simulink model "Experiment2JessDelPath_cs"  (Simulink 9.0)
settings: Solver=ode5  StartTime=0.0  StopTime=inf  FixedStep=1/300  RelTol=1e-3
PreLoadFcn:
  | mbxruntime.callbacks.PreLoadFcn(bdroot);
PostLoadFcn:
  | mbxruntime.callbacks.PostLoadFcn(bdroot);
InitFcn:
  | mbxruntime.callbacks.InitFcn(bdroot);
StartFcn:
  | mbxruntime.callbacks.StartFcn(bdroot);
StopFcn:
  | mbxruntime.callbacks.StopFcn(bdroot);
undefined symbols (not defined in the file or in its folder): DiscIntNeverNeededParam, InitImageOutputDir
libraries: PreScanSimulinkLibrary x84, simulink x43, simulink_extras x20, dspnetwork x2, vrlib x1
(part 14 of 14)

== system Experiment2JessDelPath_cs/Audi_A8_Sedan_1/Dynamics_Simple_3D/Chassis/Bicycle_model_[XYZ]/RoadContact/RoadGeometry/zRR_lowerpenetrationdetph ==
  penetrationdepth : Inport
  position_z : Inport  Port=2
  normal_z : Inport  Port=3
  Add : Sum  Inputs=-+
  Configurable Subsystem : Subsystem  BlockChoice=Discrete Transfer Fcn  mask{ComputationMode=ComputationMode}
      mask prompts: ComputationMode "Compuation mode:"
      mask init:
      | SetComputationMode(gcb,ComputationMode);
      settings: AttributesFormatString=%<BlockChoice>  OpenFcn=BringToFront(gcb);  MemberBlocks=Discrete Transfer Fcn,Transfer Fcn
      settings: TemplateBlock=|
      | PreScanSimulinkLibrary/Configurable Subsystems/TransferFunction
      | lowerpenetrationdetph/Configurable
      | Subsystem
  Constant : Constant  Value=Inf
  Constant1 : Constant  Value=-6
  Constant2 : Constant  Value=-Inf
  Data Type Conversion : DataTypeConversion  OutDataTypeStr=double
  MinMax : MinMax
  Product : Product  RndMeth=Zero
  Product1 : Product  Inputs=/*  RndMeth=Zero
  Product2 : Product  RndMeth=Zero
  Rate Limiter Dynamic : simulink/Discontinuities/Rate Limiter Dynamic
      settings: SourceProductName=Simulink
  Relational Operator : RelationalOperator  Operator===  OutDataTypeStr=boolean  RndMeth=Nearest
  Sum of Elements : Sum  Inputs=+
  Sum of Elements1 : Sum  Inputs=+
  Sum of Elements2 : Sum  Inputs=+
  Switch : Switch
  z : Outport
  wires:
  Configurable Subsystem/1(Out1) -> z/1
  Rate Limiter Dynamic/1 -> Configurable Subsystem/1(In1)
  Switch/1 -> Rate Limiter Dynamic/3
  Constant2/1 -> Switch/3
  Constant1/1 -> Switch/1
  Sum of Elements2/1 -> Switch/2
  Constant/1 -> Rate Limiter Dynamic/1
  Product1/1 -> Rate Limiter Dynamic/2
  position_z/1 -> Add/2
  Product2/1 -> Add/1
  Sum of Elements/1 -> Product1/2
  Sum of Elements1/1 -> Product1/1
  Relational Operator/1 -> Data Type Conversion/1
  Product/1 -> Sum of Elements/1
  MinMax/1 -> Relational Operator/2
  penetrationdepth/1 -> Sum of Elements2/1, Relational Operator/1, MinMax/1, Product2/1
  Add/1 -> Product/2
  normal_z/1 -> Product2/2
  Data Type Conversion/1 -> Sum of Elements1/1, Product/1

== system Experiment2JessDelPath_cs/Audi_A8_Sedan_1/Dynamics_Simple_3D/Chassis/Bicycle_model_[XYZ]/RoadContact/RoadGeometry/zRR_tyreinfo ==
  In1 : Inport
  Bus Selector2 : BusSelector  OutputSignals=TireRR.cp0.penetrationdepth,TireRR.cp1.penetrationdepth,TireRR.cp2.penetrationdepth,TireRR.cp3.penetrationdepth,TireRR.cp0.position.z,TireRR.cp1.position.z,TireRR.cp2.position.z,TireRR.cp3.position.z,TireRR.cp0.normal.z,TireRR.cp1.normal.z,TireRR.cp2.normal.z,TireRR.cp3.normal.z
  Mux11 : Mux
  Mux12 : Mux
  Mux13 : Mux
  penetrationdepth : Outport
  position_z : Outport  Port=2
  normal_z : Outport  Port=3
  wires:
  Mux13/1 -> normal_z/1
  Mux12/1 -> position_z/1
  Mux11/1 -> penetrationdepth/1
  In1/1 -> Bus Selector2/1
  Bus Selector2/12 -> Mux13/4  "<z>"
  Bus Selector2/11 -> Mux13/3  "<z>"
  Bus Selector2/10 -> Mux13/2  "<z>"
  Bus Selector2/9 -> Mux13/1  "<z>"
  Bus Selector2/8 -> Mux12/4  "<z>"
  Bus Selector2/7 -> Mux12/3  "<z>"
  Bus Selector2/6 -> Mux12/2  "<z>"
  Bus Selector2/5 -> Mux12/1  "<z>"
  Bus Selector2/4 -> Mux11/4  "<penetrationdepth>"
  Bus Selector2/3 -> Mux11/3  "<penetrationdepth>"
  Bus Selector2/2 -> Mux11/2  "<penetrationdepth>"
  Bus Selector2/1 -> Mux11/1  "<penetrationdepth>"

== system Experiment2JessDelPath_cs/Audi_A8_Sedan_1/Dynamics_Simple_3D/Chassis/Bicycle_model_[XYZ]/X_Motion/Max RPM and zero- velocity detection/Configurable Subsystem ==
  Discrete Step : Step  Time=0.0001  Before=1  After=0  SampleTime=TimeStep
  Out1 : Outport
  wires:
  Discrete Step/1 -> Out1/1

== system Experiment2JessDelPath_cs/Audi_A8_Sedan_1/Dynamics_Simple_3D/Chassis/Bicycle_model_[XYZ]/X_Motion/Max RPM and zero- velocity detection/SR-Memory ==
  Signal : Inport
  Set : Inport  Port=2
  Reset : Inport  Port=3
  Constant : Constant  Value=0
  Detect Rise Positive : simulink/Logic and Bit Operations/Detect Rise Positive  vinit=0  InputProcessing=Inherited  OutDataTypeStr=uint8
  Detect Rise Positive1 : simulink/Logic and Bit Operations/Detect Rise Positive  vinit=0  InputProcessing=Inherited  OutDataTypeStr=uint8
  Manual Switch : ManualSwitch
  Manual Switch1 : ManualSwitch
  Switch : Switch  Criteria=u2 ~= 0
  Switch1 : Switch  Criteria=u2 ~= 0
  Unit Delay : UnitDelay  SampleTime=-1
  Out : Outport
  wires:
  Manual Switch/1 -> Switch/2
  Detect Rise Positive/1 -> Manual Switch/1
  Set/1 -> Manual Switch/2, Detect Rise Positive/1
  Unit Delay/1 -> Switch/3
  Signal/1 -> Switch/1
  Detect Rise Positive1/1 -> Manual Switch1/1
  Reset/1 -> Detect Rise Positive1/1, Manual Switch1/2
  Manual Switch1/1 -> Switch1/2
  Switch1/1 -> Out/1, Unit Delay/1
  Switch/1 -> Switch1/3
  Constant/1 -> Switch1/1

== system Experiment2JessDelPath_cs/Audi_A8_Sedan_1/PreScan_Contact_Sensor/Vehicle Local to World/state2FullState/limit roll/Substitute 90 & 270 deg (and its plurals)/Angle 0-360 deg limiter ==
  Angle [deg] : Inport
  Gain : Gain  Gain=1/360
  Gain1 : Gain  Gain=360
  Rounding Function : Rounding
  Sum : Sum  Inputs=|-+
  LimAngle [deg] : Outport
  wires:
  Gain/1 -> Rounding Function/1
  Rounding Function/1 -> Gain1/1
  Gain1/1 -> Sum/1
  Angle [deg]/1 -> Gain/1, Sum/2
  Sum/1 -> LimAngle [deg]/1

== system Experiment2JessDelPath_cs/Audi_A8_Sedan_1/Dynamics_Simple_3D/Chassis/Bicycle_model_[XYZ]/RoadContact/RoadGeometry/Calc_z/zC ==
  Array : Inport
  Compare To Constant : simulink/Logic and Bit Operations/Compare To Constant  relop=>  const=0  OutDataTypeStr=uint8  ZeroCross=off
  Constant : Constant  Value=NaN
  Product : Product  Inputs=*/  RndMeth=Zero
  Sum of Elements : Sum  Inputs=+
  Switch : Switch
  Width : Width
  Mean : Outport
  wires:
  Array/1 -> Sum of Elements/1, Width/1
  Sum of Elements/1 -> Product/1
  Width/1 -> Product/2, Compare To Constant/1
  Compare To Constant/1 -> Switch/2
  Product/1 -> Switch/1
  Constant/1 -> Switch/3
  Switch/1 -> Mean/1

== system Experiment2JessDelPath_cs/Audi_A8_Sedan_1/Dynamics_Simple_3D/Chassis/Bicycle_model_[XYZ]/RoadContact/RoadGeometry/zFL_lowerpenetrationdetph/Configurable Subsystem ==
  In1 : Inport
  Discrete Transfer Fcn : DiscreteTransferFcn  Numerator="[  1-exp(-( ( TimeStep ) / (1/(2*pi)) ) )  ]"  Denominator="[  1   -exp(-( ( TimeStep ) / (1/(2*pi)) ) )   ]"  SampleTime=TimeStep
  Out1 : Outport
  wires:
  In1/1 -> Discrete Transfer Fcn/1
  Discrete Transfer Fcn/1 -> Out1/1

== system Experiment2JessDelPath_cs/Audi_A8_Sedan_1/Dynamics_Simple_3D/Chassis/Bicycle_model_[XYZ]/RoadContact/RoadGeometry/zFR_lowerpenetrationdetph/Configurable Subsystem ==
  In1 : Inport
  Discrete Transfer Fcn : DiscreteTransferFcn  Numerator="[  1-exp(-( ( TimeStep ) / (1/(2*pi)) ) )  ]"  Denominator="[  1   -exp(-( ( TimeStep ) / (1/(2*pi)) ) )   ]"  SampleTime=TimeStep
  Out1 : Outport
  wires:
  In1/1 -> Discrete Transfer Fcn/1
  Discrete Transfer Fcn/1 -> Out1/1

== system Experiment2JessDelPath_cs/Audi_A8_Sedan_1/Dynamics_Simple_3D/Chassis/Bicycle_model_[XYZ]/RoadContact/RoadGeometry/zRL_lowerpenetrationdetph/Configurable Subsystem ==
  In1 : Inport
  Discrete Transfer Fcn : DiscreteTransferFcn  Numerator="[  1-exp(-( ( TimeStep ) / (1/(2*pi)) ) )  ]"  Denominator="[  1   -exp(-( ( TimeStep ) / (1/(2*pi)) ) )   ]"  SampleTime=TimeStep
  Out1 : Outport
  wires:
  In1/1 -> Discrete Transfer Fcn/1
  Discrete Transfer Fcn/1 -> Out1/1

== system Experiment2JessDelPath_cs/Audi_A8_Sedan_1/Dynamics_Simple_3D/Chassis/Bicycle_model_[XYZ]/RoadContact/RoadGeometry/zRR_lowerpenetrationdetph/Configurable Subsystem ==
  In1 : Inport
  Discrete Transfer Fcn : DiscreteTransferFcn  Numerator="[  1-exp(-( ( TimeStep ) / (1/(2*pi)) ) )  ]"  Denominator="[  1   -exp(-( ( TimeStep ) / (1/(2*pi)) ) )   ]"  SampleTime=TimeStep
  Out1 : Outport
  wires:
  In1/1 -> Discrete Transfer Fcn/1
  Discrete Transfer Fcn/1 -> Out1/1

== matlab function Audi_A8_Sedan_1/HID_Control/Custom_Control/MATLAB Function ==
  data: trustSignals input double; trustDownBtn input double; trustUpBtn input double; trust output double; trustSemantics input double
function trust = trustLogic(trustSignals, trustDownBtn, trustUpBtn, trustSemantics)

%also take in auto-mode parameter so to know when to do things

persistent currentTrust;
persistent previousTrust;
persistent lastDistrustBtn;
persistent lastTrustBtn;


if isempty(previousTrust)
    previousTrust = 0;
    currentTrust = 3;
    lastDistrustBtn = 0;
    lastTrustBtn = 0;
end

%SO INSTEAD OF ==3, TREAT AS AN ARRAY WITH THAT INDEX
%THE trustSignals INPUT IS ACTUALLY AN ARRAY. WE NEED TO FIX DAT
%FIGURE OUT HOW BUTTON 2 OR 3 IS REPRESENTED IN THE ARRAY AS INPUT

for i=1:length(trustSignals)
    if trustSignals(i) && ~previousTrust(i)
        % If any of the gear signals is enabled, use its semantic
        currentTrust = trustSemantics(i); 
        break;
    elseif previousTrust(i) && ~trustSignals(i)
        % If any of the gear signals is disabled, set gear to 0
        currentTrust = 0; 
    end
end

% Trust adjust is a must
if (trustSignals == 3) && ~lastDistrustBtn
    currentTrust = currentTrust - 1;
end
if (trustSignals == 2) && ~lastTrustBtn
    currentTrust = currentTrust + 1;
end

% Cap the Trust between 1-5

currentTrust = min(max(minTrust));
% Store statest, currentTrust), maxTrust);

previousTrust = currentTrust;
lastDistrustBtn = (trustSignals == 3);
lastTrustBtn = (trustSignals == 2);



trust = double(currentTrust);

== matlab function Audi_A8_Sedan_1/HID_Control/Custom_Control/Gear Button Logic ==
  data: gear output double; gearButtonSignals input double; gearSemantics input double; shiftDownBtn input double; shiftUpBtn input double
function gear = gearButtonLogic(gearButtonSignals, gearSemantics, shiftDownBtn, shiftUpBtn)
%eml

% example signals for 1 frame:
%gearButtonSignals = [  0 0 1 0 0 0 0 ];
%    gearSemantics = [ -1 1 2 3 4 5 6 ];

% persistent values are use to inspect changes in the signals
persistent currentGear;
persistent previousGearSignals;
persistent lastShiftDownBtn;
persistent lastshiftUpBtn;

% Write values for the first run
if isempty(previousGearSignals)
    previousGearSignals = zeros(size(gearButtonSignals));
    currentGear = 0;
    lastShiftDownBtn = 0;
    lastshiftUpBtn = 0;
end

% Gear setting logic
for i=1:length(gearButtonSignals)
    if gearButtonSignals(i) && ~previousGearSignals(i)
        % If any of the gear signals is enabled, use its semantic
        currentGear = gearSemantics(i); 
        break;
    elseif previousGearSignals(i) && ~gearButtonSignals(i)
        % If any of the gear signals is disabled, set gear to 0
        currentGear = 0; 
    end
end

% Gear shifting logic
if shiftDownBtn && ~lastShiftDownBtn
    currentGear = currentGear - 1;
end
if shiftUpBtn && ~lastshiftUpBtn
    currentGear = currentGear + 1;
end

% Cap the gear between [minGear, maxGear]
minGear = min(gearSemantics);
maxGear = max(gearSemantics);
currentGear = min(max(minGear, currentGear), maxGear);

% Store states
previousGearSignals = gearButtonSignals;
lastShiftDownBtn = shiftDownBtn;
lastshiftUpBtn = shiftUpBtn;

gear = double(currentGear);
